simulink model "MotorCtrl_MILS"  (R2018b)
settings: configuration reference "Config_Plant" (kept outside this file)
settings Model: Creator=E00026  LastModifiedBy=E00026
settings ConfigSetRef: SourceLocation=Base Workspace

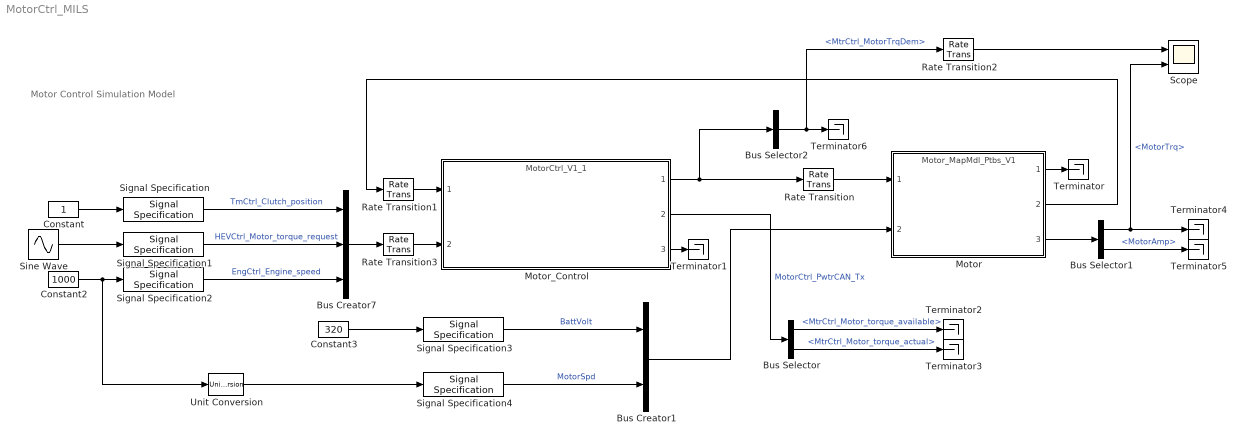
== system MotorCtrl_MILS ==
  note: Motor Control Simulation Model
  Bus Creator1 : BusCreator  Inputs=2
  Bus Creator7 : BusCreator  Inputs=3
  Bus Selector : BusSelector  OutputSignals=MtrCtrl_Motor_torque_available,MtrCtrl_Motor_torque_actual
  Bus Selector1 : BusSelector  OutputSignals=MotorTrq,MotorAmp
  Bus Selector2 : BusSelector  OutputSignals=MtrCtrl_MotorTrqDem
  Constant : Constant
  Constant2 : Constant  Value=1000
  Constant3 : Constant  Value=320
  Motor : ModelReference  ModelNameDialog=Motor_MapMdl_Ptbs_V1  SimulationMode=Normal  ModelReferenceVersion=1.1342
  Motor_Control : ModelReference  ModelNameDialog=MotorCtrl_V1_1.slx  SimulationMode=Normal  ModelReferenceVersion=1.0.23
  Rate Transition{,1..3} (4 alike) : RateTransition  Deterministic=off
  Scope : Scope  NumInputPorts=2
  Signal Specification{,1..4} (5 alike) : SignalSpecification
  Sine Wave : Sin  Amplitude=10  Bias=5  Frequency=0.05  SampleTime=0
  Terminator{,1..6} (7 alike) : Terminator
  Unit Conversion : UnitConversion
  wires:
  Motor_Control/1 -> Bus Selector2/1, Rate Transition/1
  Motor/1 -> Terminator/1
  Motor_Control/2 -> Bus Selector/1  "MotorCtrl_PwtrCAN_Tx"
  Bus Creator7/1 -> Rate Transition3/1
  Signal Specification/1 -> Bus Creator7/1  "TmCtrl_Clutch_position"
  Signal Specification2/1 -> Bus Creator7/3  "EngCtrl_Engine_speed"
  Signal Specification1/1 -> Bus Creator7/2  "HEVCtrl_Motor_torque_request"
  Constant/1 -> Signal Specification/1
  Sine Wave/1 -> Signal Specification1/1
  Motor_Control/3 -> Terminator1/1
  Bus Selector/1 -> Terminator2/1  "<MtrCtrl_Motor_torque_available>"
  Bus Selector/2 -> Terminator3/1  "<MtrCtrl_Motor_torque_actual>"
  Motor/3 -> Bus Selector1/1
  Bus Selector1/1 -> Scope/2, Terminator4/1  "<MotorTrq>"
  Bus Selector1/2 -> Terminator5/1  "<MotorAmp>"
  Constant2/1 -> Unit Conversion/1, Signal Specification2/1
  Constant3/1 -> Signal Specification3/1
  Signal Specification4/1 -> Bus Creator1/2  "MotorSpd"
  Signal Specification3/1 -> Bus Creator1/1  "BattVolt"
  Bus Creator1/1 -> Motor/2
  Bus Selector2/1 -> Rate Transition2/1, Terminator6/1  "<MtrCtrl_MotorTrqDem>"
  Rate Transition/1 -> Motor/1
  Motor/2 -> Rate Transition1/1
  Rate Transition2/1 -> Scope/1
  Rate Transition3/1 -> Motor_Control/2
  Rate Transition1/1 -> Motor_Control/1
  Unit Conversion/1 -> Signal Specification4/1
